simulink model "DriveAround"  (R2021b)
settings: Solver=FixedStepAuto  StartTime=0.0  StopTime=inf  FixedStep=0.02  RelTol=1e-3  EnableMultiTasking=on
InitFcn:
  | InitFcn;
values from neighbouring files (symbols this model uses):
  desiredSpeed = -.5    (= -0.5)    [InitFcn.m]
  LookDistance = 0.4    [InitFcn.m]
  vehicleDynamics = [b1 L1 L2 b2]    [InitFcn.m]
  X_waypoints = linspace(-L2,-15,15000)    [InitFcn.m]
  Y_waypoints = (sin(X_waypoints+L2+pi/2+0.1)-1)*magnitude    [InitFcn.m]
libraries: arduinolib x4
settings Model: ExtModeTrigDuration=2  Creator=anton  LastModifiedBy=vikto
settings SolverCC: AlgebraicLoopSolver=TrustRegion
settings OptimizationCC: EnhancedBackFolding=on  PassReuseOutputArgsThreshold=0  MaxStackSize=64  OptimizeBlockOrder=speed  DifferentSizesBufferReuse=on  OptimizationCustomize=off
settings DebuggingCC: ParameterTunabilityLossMsg=error  SFMachineParentedDataDiag=warning
settings HardwareCC: ProdBitPerPointer=32  ProdBitPerSizeT=32  ProdBitPerPtrDiffT=32  ProdLargestAtomicInteger=Long  ProdLargestAtomicFloat=Double  ProdWordSize=32  ProdHWDeviceType=ARM Compatible->ARM Cortex  UseEmbeddedCoderFeatures=off  UseSimulinkCoderFeatures=off
settings SFSimCC: MATLABDynamicMemAlloc=off
settings RTWCC: Description=Embedded Coder  SystemTargetFile=ert.tlc  HardwareBoard=Arduino Due  TemplateMakefile=ert_default_tmf  Toolchain=Arduino ARM  BuildConfiguration=Faster Runs
settings CodeAppCC: ForceParamTrailComments=on  OperatorAnnotations=on
settings ERTTargetCC: ERTCustomFileBanners=off  SupportContinuousTime=on  SupportNonInlinedSFcns=on  RemoveResetFunc=off  SupportVariableSizeSignals=on  ModelStepFunctionPrototypeControlCompliant=off  ExtModeTransport=3  ExtModeStaticAlloc=on  ExtModeStaticAllocSize=24576  ExtModeMexFile=ext_xcp  ExtModeIntrfLevel=Level2 - Open

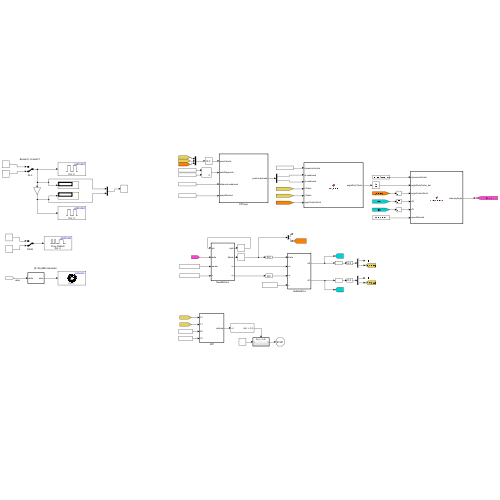
[thumbnail: Simulink's stored preview of the top-level diagram]
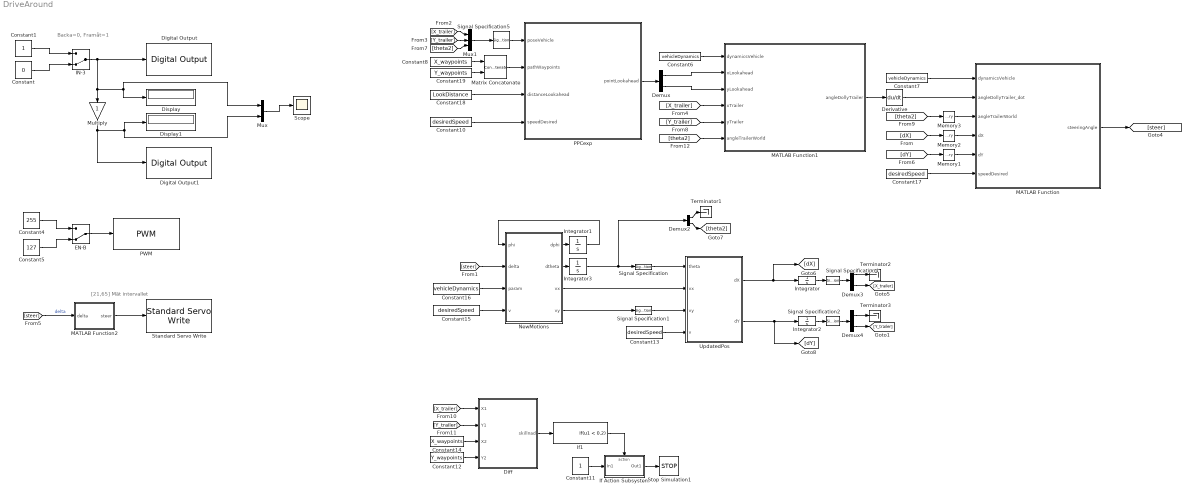
== system DriveAround ==
  note: [21,65] Mät intervallet
  note: Backa=0, Framåt=1
  Constant : Constant  Value=0
  Constant1 : Constant
  Constant{10,13,15,17} (4 alike) : Constant  Value=desiredSpeed
  Constant11 : Constant
  Constant12 : Constant  Value=Y_waypoints
  Constant14 : Constant  Value=X_waypoints
  Constant16 : Constant  Value=vehicleDynamics
  Constant18 : Constant  Value=LookDistance
  Constant19 : Constant  Value=Y_waypoints
  Constant4 : Constant  Value=255
  Constant5 : Constant  Value=127
  Constant6 : Constant  Value=vehicleDynamics
  Constant7 : Constant  Value=vehicleDynamics
  Constant8 : Constant  Value=X_waypoints
  Demux{,2..4} (4 alike) : Demux  Outputs=2
  Derivative : Derivative
  Diff : MATLAB Function  TreatAsAtomicUnit=on
  Digital Output : arduinolib/Digital Output  pinNumber=2  Direction=output  blockPlatform=arduino
  Digital Output1 : arduinolib/Digital Output  pinNumber=3  Direction=output  blockPlatform=arduino
  Display : Display
  Display1 : Display
  EN-B : ManualSwitch  CurrentSetting=0
  IN-3 : ManualSwitch  CurrentSetting=0
  If Action Subsystem : Subsystem  TreatAsAtomicUnit=on
  If1 : If  IfExpression=u1 < 0.2  ShowElse=off
  Integrator : Integrator  InitialCondition=[0;-1.3]
  Integrator1 : Integrator
  Integrator2 : Integrator
  Integrator3 : Integrator
  MATLAB Function : MATLAB Function  TreatAsAtomicUnit=on
  MATLAB Function1 : MATLAB Function  TreatAsAtomicUnit=on
  MATLAB Function2 : MATLAB Function  TreatAsAtomicUnit=on
  Matrix Concatenate : Concatenate  Mode=Multidimensional array  ConcatenateDimension=2
  Memory1 : Memory
  Memory2 : Memory
  Memory3 : Memory
  Multiply : Gain
  Mux : Mux  Inputs=2
  Mux1 : Mux  Inputs=3
  NewMotions : MATLAB Function  TreatAsAtomicUnit=on
  PPCexp : MATLAB Function  TreatAsAtomicUnit=on
  PWM : arduinolib/PWM  pinNumber=4  frequencyType=Default  desiredFrequency=490.2  achievableFrequency=490.2
  Scope : Scope
  Signal Specification{,1..2,4} (4 alike) : SignalSpecification  Dimensions=2
  Signal Specification5 : SignalSpecification  Dimensions=3
  Standard Servo Write : arduinolib/Standard Servo Write  pinNumber=11  ServoIndex=0  blockPlatform=arduino
      settings: SourceProductName=Simulink Support Package for Arduino Hardware
  Stop Simulation1 : Stop
  Terminator1 : Terminator
  Terminator2 : Terminator
  Terminator3 : Terminator
  UpdatedPos : MATLAB Function  TreatAsAtomicUnit=on
  wires:
  Constant1/1 -> IN-3/1
  Constant5/1 -> EN-B/2
  Mux/1 -> Scope/1
  EN-B/1 -> PWM/1
  IN-3/1 -> Digital Output/1, Multiply/1, Display/1, Mux/1
  Constant4/1 -> EN-B/1
  Constant/1 -> IN-3/2
  [dY] -> Memory1/1
  Signal Specification4/1 -> Demux3/1
  If1/1 -> If Action Subsystem/Action
  NewMotions/1(dphi) -> Integrator1/1
  Constant14/1 -> Diff/3(X2)
  Constant11/1 -> If Action Subsystem/1(In1)
  Demux/2 -> MATLAB Function1/3(yLookahead)
  Signal Specification5/1 -> PPCexp/1(poseVehicle)
  NewMotions/4(vy) -> Signal Specification1/1
  UpdatedPos/1(dX) -> Integrator/1, [dX]
  [X_trailer] -> Diff/1(X1)
  If Action Subsystem/1(Out1) -> Stop Simulation1/1
  NewMotions/2(dtheta) -> Integrator3/1
  [Y_trailer] -> Diff/2(Y1)
  Constant12/1 -> Diff/4(Y2)
  Demux2/2 -> [theta2]
  Mux1/1 -> Signal Specification5/1
  [X_trailer] -> MATLAB Function1/4(xTrailer)
  NewMotions/3(vx) -> UpdatedPos/2(vx)
  Demux2/1 -> Terminator1/1
  Signal Specification2/1 -> Demux4/1
  [steer] -> NewMotions/2(delta)
  MATLAB Function1/1(angleDollyTrailer) -> Derivative/1
  Derivative/1 -> MATLAB Function/2(angleDollyTrailer_dot)
  [theta2] -> MATLAB Function1/6(angleTrailerWorld)
  Demux3/2 -> [X_trailer]
  Demux4/2 -> [Y_trailer]
  Diff/1(skillnad) -> If1/1
  Matrix Concatenate/1 -> PPCexp/2(pathWaypoints)
  MATLAB Function/1(steeringAngle) -> [steer]
  Constant13/1 -> UpdatedPos/4(v)
  Signal Specification/1 -> UpdatedPos/1(theta)
  Integrator3/1 -> Demux2/1, Signal Specification/1
  Integrator/1 -> Signal Specification4/1
  Demux/1 -> MATLAB Function1/2(xLookahead)
  [theta2] -> Mux1/3
  Memory1/1 -> MATLAB Function/5(dY)
  PPCexp/1(pointLookahead) -> Demux/1
  [Y_trailer] -> Mux1/2
  Integrator2/1 -> Signal Specification2/1
  [X_trailer] -> Mux1/1
  Signal Specification1/1 -> UpdatedPos/3(vy)
  [Y_trailer] -> MATLAB Function1/5(yTrailer)
  [steer] -> MATLAB Function2/1(delta)  "delta"
  MATLAB Function2/1(steer) -> Standard Servo Write/1
  Demux3/1 -> Terminator2/1
  Demux4/1 -> Terminator3/1
  Constant15/1 -> NewMotions/4(v)
  Constant16/1 -> NewMotions/3(param)
  Integrator1/1 -> NewMotions/1(phi)
  [dX] -> Memory2/1
  Memory2/1 -> MATLAB Function/4(dX)
  [theta2] -> Memory3/1
  Memory3/1 -> MATLAB Function/3(angleTrailerWorld)
  Constant17/1 -> MATLAB Function/6(speedDesired)
  Constant10/1 -> PPCexp/4(speedDesired)
  Constant18/1 -> PPCexp/3(distanceLookahead)
  Constant8/1 -> Matrix Concatenate/1
  Constant19/1 -> Matrix Concatenate/2
  Constant6/1 -> MATLAB Function1/1(dynamicsVehicle)
  UpdatedPos/2(dY) -> [dY], Integrator2/1
  Constant7/1 -> MATLAB Function/1(dynamicsVehicle)
  Multiply/1 -> Display1/1, Mux/2, Digital Output1/1

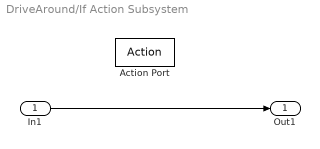
== system DriveAround/If Action Subsystem ==
  In1 : Inport
  Action Port : ActionPort  ActionPortLabel=if(u1 < 0.2)
  Out1 : Outport
  wires:
  In1/1 -> Out1/1

== matlab function DriveAround/MATLAB Function2 ==
  data: delta input; steer output
function steer = deltatosteer(delta)
    steer=delta*21.5*180/(27*pi)+43; %halva intervallet=21.5, mittpunkten=43.
end

== matlab function DriveAround/PPCexp ==
  data: poseVehicle input; pointLookahead output; pathWaypoints input; distanceLookahead input; speedDesired input
function pointLookahead  = PurePursuit(poseVehicle, pathWaypoints, distanceLookahead, speedDesired)
    controller = controllerPurePursuit('DesiredLinearVelocity', abs(speedDesired), 'Waypoints', pathWaypoints, 'LookaheadDistance', distanceLookahead);
    [vel, angvel, pointLookahead] = controller(poseVehicle);
end

== matlab function DriveAround/NewMotions ==
  data: phi input; dphi output; delta input; param input; dtheta output; vx output; vy output; v input
%This function is our "Plant" in here is all the kinematics of trailer and
%dolly. It output is change in phi and theta and velocity in x and y
%direction. Most of this is taken from the previous code but change in
%varibale names
function [dphi, dtheta, vx,vy] = Motions(phi, delta, param, v)
    b_d = param(1); % Length from rear-axle to center of dolly
    L_d = param(2); % Length of between wheels dolly
    L_s = param(3); % Length between wheelbase and connection of trailer
    b_s = param(4); % Trailer slip of

    dphi = 0;         % Hitch angle at point A    
    dtheta = [0;0];     % Change in yaw angles
    vx = 0;           % Longitudinal velocity
    vy=[0;0];

    %dolly
    dtheta(1) =(v/L_d)*tan(delta); %yaw rate of the tractor [rad/s]
    vy(1) = b_d*dtheta(1);       % Lateral velocity at point A
    
    %släp
    dtheta(2) =(1/L_s)*(-v*sin(phi) + cos(phi)*vy(1)); %Yaw rate of trailer 1 [rad/s]
    vx = v * cos(phi)+ vy(1)*sin(phi); % longitudinal velocity at point B
    vy(2) = -dtheta(2)*b_s; % Lateral velocity at point B
    dphi = dtheta(2) - dtheta(1); %Articulation angle rate at pivot 1 [rad/s]
end

== matlab function DriveAround/UpdatedPos ==
  data: theta input; dX output; vx input; vy input; v input; dY output
function [dX,dY]  = PosGlobal(theta, vx, vy, v)
    dX=[0;0];
    dX(1) = v*cos(theta(1))-vy(1)*sin(theta(1));
    dX(2) = vx*cos(theta(2))-vy(2)*sin(theta(2));

    dY=[0;0];
    dY(1) = vy(1)*cos(theta(1))+v*sin(theta(1));
    dY(2) = vy(2)*cos(theta(2))+vx*sin(theta(2));  
end

== matlab function DriveAround/Diff ==
  data: X1 input; skillnad output; Y1 input; X2 input; Y2 input
function skillnad = diffunktion(X1,Y1,X2,Y2)
trailer=[X1 Y1];
path=[X2(end) Y2(end)];
skillnad=norm(path-trailer);
end

== matlab function DriveAround/MATLAB Function ==
  data: dynamicsVehicle input; angleDollyTrailer_dot input; steeringAngle output; angleTrailerWorld input; dX input; dY input; speedDesired input
%This function is supposed to calculate a desired steeringangle so that
%phi_des is meet. 
function steeringAngle = WheelAngle(dynamicsVehicle, angleDollyTrailer_dot, angleTrailerWorld, dX, dY, speedDesired)
    b_d = dynamicsVehicle(1);
    L_d = dynamicsVehicle(2);
    L_s = dynamicsVehicle(3);
    b_s = dynamicsVehicle(4);
    
    dtheta2 = (dX(1) * sin(angleTrailerWorld) - dY(1) * cos(angleTrailerWorld)) / L_s;
    steeringAngle = -atan((dtheta2 - angleDollyTrailer_dot) * L_d / speedDesired);
end

== matlab function DriveAround/MATLAB Function1 ==
  data: dynamicsVehicle input; angleDollyTrailer output; xLookahead input; yLookahead input; xTrailer input; yTrailer input; angleTrailerWorld input
%this funciton calculates phi_error which is the diffrence of angle between
%theta (trailers position angle) and the lookahead point (desired heading 
%angle). Which gives us phi_des, desired angle between trailer and dolly
function angleDollyTrailer = DollyAngle(dynamicsVehicle, xLookahead, yLookahead, xTrailer, yTrailer, angleTrailerWorld)
    b_d = dynamicsVehicle(1); % make struct instead
    L_d = dynamicsVehicle(2);
    trailerLength = dynamicsVehicle(3);
    b_s = dynamicsVehicle(4);

    deltaX = xTrailer - xLookahead;
    deltaY = yTrailer - yLookahead;
    XY_diff = sqrt(deltaX^2 + deltaY^2);

    % använd atan2 istället? atan2(deltaY, deltaX) - angleTrailerWorld;
    % kanske behöver invertera deltaX och deltaY.
    theta2_err = acos(deltaX / XY_diff) - angleTrailerWorld;

    if deltaY < 0     %för att den ska gå varvet runt, klarar dock bara 3/4,verkar bero på waypoints
        theta2_err = pi + acos(-deltaX / XY_diff) - angleTrailerWorld;
    end

    angleDollyTrailer = -3 * atan2(2 * trailerLength * sin(theta2_err), XY_diff);
end
